simulink subsystem "Controller_Sub"  (R2024a)
settings: Solver=VariableStepAuto  StartTime=0.0  StopTime=10.0  RelTol=1e-3
undefined symbols (not defined in the file): body_inertia, body_mass, Dinv, DiscIntNeverNeededParam, Dmat, motor_gyration, motor_resistance, nominal_voltage, pwm_limit, torque_limit, wheel_distance, wheel_radius
libraries: slpidlib x2, dspfdesign x2
settings Model: Creator=Marij  LastModifiedBy=Marij

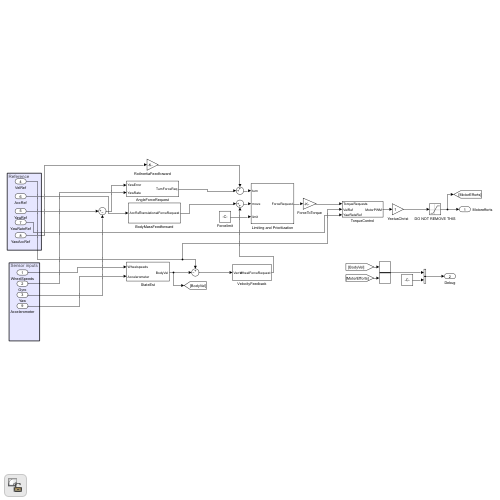
[thumbnail: Simulink's stored preview of the top-level diagram]
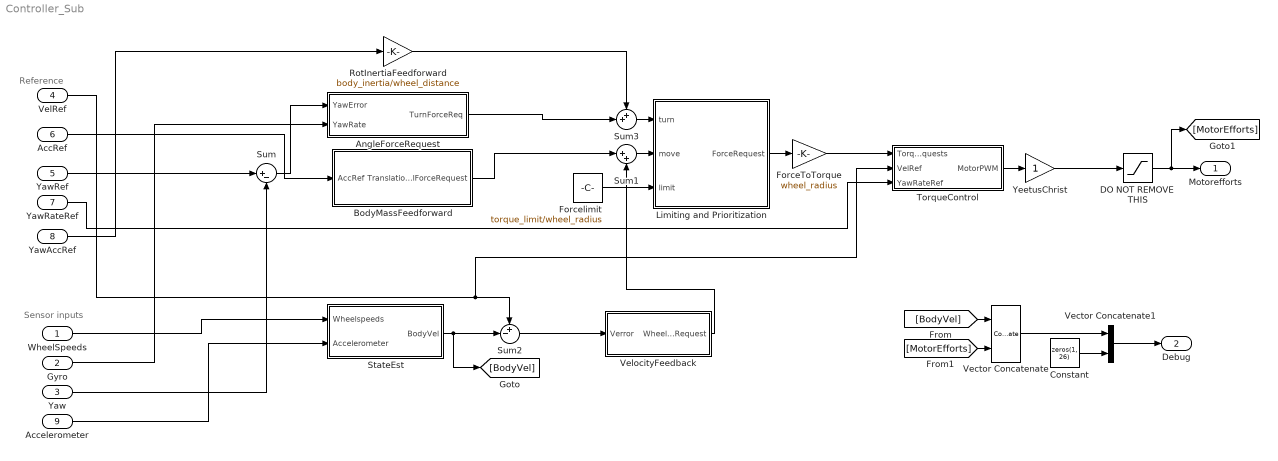
== system Controller_Sub ==
  note: Reference
  note: Sensor inputs
  WheelSpeeds : Inport  OutDataTypeStr=single  Unit=rad/s  PortDimensions=4  LockScale=on
  Gyro : Inport  Port=2  OutDataTypeStr=single  Unit=rad/s  PortDimensions=1
  Yaw : Inport  Port=3  OutDataTypeStr=single  Unit=rad  PortDimensions=1
  VelRef : Inport  Port=4  OutDataTypeStr=single  Unit=m/s  PortDimensions=2
  YawRef : Inport  Port=5
  AccRef : Inport  Port=6  OutDataTypeStr=single  Unit=m/s^2  PortDimensions=2
  YawRateRef : Inport  Port=7  OutDataTypeStr=single  Unit=rad/s
  YawAccRef : Inport  Port=8  OutDataTypeStr=single  Unit=rad/s^2
  Accelerometer : Inport  Port=9  OutDataTypeStr=single  Unit=m/s^2  PortDimensions=2
  AngleForceRequest : Subsystem
  BodyMassFeedforward : Subsystem
  Constant : Constant  Value=zeros(1, 26)  OutDataTypeStr=single
  DO NOT REMOVE THIS : Saturate  UpperLimit=pwm_limit  LowerLimit=-pwm_limit
  ForceToTorque : Gain  Gain=wheel_radius
  Forcelimit : Constant  Value=torque_limit/wheel_radius
  Limiting and Prioritization : Subsystem
  RotInertiaFeedforward : Gain  Gain=body_inertia/wheel_distance
  StateEst : Subsystem
  Sum : Sum  Inputs=|+-
  Sum1 : Sum  Inputs=|++
  Sum2 : Sum  Inputs=+-|
  Sum3 : Sum  Inputs=++|
  TorqueControl : Subsystem
  Vector Concatenate : Concatenate
  Vector Concatenate1 : Concatenate
  VelocityFeedback : Subsystem
  YeetusChrist : Gain
  Motorefforts : Outport  OutDataTypeStr=single  PortDimensions=4
  Debug : Outport  Port=2  OutDataTypeStr=single  PortDimensions=32
  wires:
  YeetusChrist/1 -> DO NOT REMOVE THIS/1
  Gyro/1 -> AngleForceRequest/2(YawRate)
  AccRef/1 -> BodyMassFeedforward/1(AccRef)
  Sum/1 -> AngleForceRequest/1(YawError)
  Accelerometer/1 -> StateEst/2(Accelerometer)
  StateEst/1(BodyVel) -> Sum2/2, [BodyVel]
  Sum3/1 -> Limiting and Prioritization/1(turn)
  YawRef/1 -> Sum/1
  TorqueControl/1(MotorPWM) -> YeetusChrist/1
  WheelSpeeds/1 -> StateEst/1(Wheelspeeds)
  Limiting and Prioritization/1(ForceRequest) -> ForceToTorque/1
  DO NOT REMOVE THIS/1 -> [MotorEfforts], Motorefforts/1
  Sum2/1 -> VelocityFeedback/1(Verror)
  [BodyVel] -> Vector Concatenate/1
  Yaw/1 -> Sum/2
  RotInertiaFeedforward/1 -> Sum3/1
  [MotorEfforts] -> Vector Concatenate/2
  VelocityFeedback/1(WheelForceRequest) -> Sum1/2
  Vector Concatenate1/1 -> Debug/1
  YawAccRef/1 -> RotInertiaFeedforward/1
  Vector Concatenate/1 -> Vector Concatenate1/1
  VelRef/1 -> TorqueControl/2(VelRef), Sum2/1
  BodyMassFeedforward/1(TranslationalForceRequest) -> Sum1/1
  YawRateRef/1 -> TorqueControl/3(YawRateRef)
  AngleForceRequest/1(TurnForceReq) -> Sum3/2
  ForceToTorque/1 -> TorqueControl/1(TorqueRequests)
  Sum1/1 -> Limiting and Prioritization/2(move)
  Constant/1 -> Vector Concatenate1/2
  Forcelimit/1 -> Limiting and Prioritization/3(limit)

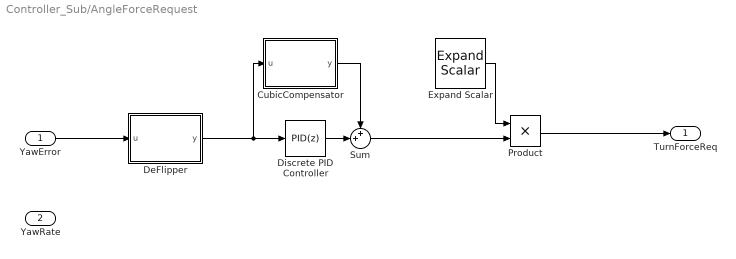
== system Controller_Sub/AngleForceRequest ==
  YawError : Inport  Unit=rad
  YawRate : Inport  Port=2
  CubicCompensator : MATLAB Function  TreatAsAtomicUnit=on
  DeFlipper : MATLAB Function  TreatAsAtomicUnit=on
  Discrete PID Controller : slpidlib/PID Controller  Controller=PID  Form=Parallel  TimeDomain=Discrete-time  UseExternalTs=off  SampleTime=-1  IntegratorMethod=Trapezoidal  FilterMethod=Trapezoidal  ControllerParametersSource=internal  P=9.0  I=0.1  UseKiTs=off  D=0.8  UseExternalDerivativeSource=off  N=100  UseFilter=on  TunerSelectOption=Transfer Function Based (PID Tuner App)  InitialConditionSource=internal  InitialConditionForIntegrator=0  InitialConditionForFilter=0  DifferentiatorICPrevScaledInput=0  ExternalReset=none  TrackingMode=off  Kt=1  LimitOutput=off  SatLimitsSource=internal  UpperSaturationLimit=inf  LowerSaturationLimit=-inf  LinearizeAsGain=off  AntiWindupMode=none  Kb=1  LimitIntegrator=off  UpperIntegratorSaturationLimit=inf  LowerIntegratorSaturationLimit=-inf  POutMin=[]  POutMax=[]  IOutMin=[]  IOutMax=[]  DOutMin=[]  DOutMax=[]  NOutMin=[]  NOutMax=[]  SumOutMin=[]  SumOutMax=[]  SaturationOutMin=[]  SaturationOutMax=[]  PParamMin=[]  PParamMax=[]  IParamMin=[]  IParamMax=[]  DParamMin=[]  DParamMax=[]  NParamMin=[]  NParamMax=[]  KbParamMin=[]  KbParamMax=[]  KtParamMin=[]  KtParamMax=[]  KbOutMin=[]  KbOutMax=[]  KtOutMin=[]  KtOutMax=[]  IntegratorOutMin=[]  IntegratorOutMax=[]  FilterOutMin=[]  FilterOutMax=[]  SumI1OutMin=[]  SumI1OutMax=[]  SumI2OutMin=[]  SumI2OutMax=[]  SumI3OutMin=[]  SumI3OutMax=[]  SumI4OutMin=[]  SumI4OutMax=[]  SumDOutMin=[]  SumDOutMax=[]  DifferentiatorOutMin=[]  DifferentiatorOutMax=[]  FilterDiffOutCoefMin=[]  FilterDiffOutCoefMax=[]  ReciprocalOutMin=[]  ReciprocalOutMax=[]  SumDenOutMin=[]  SumDenOutMax=[]  SumNumOutMin=[]  SumNumOutMax=[]  DivideOutMin=[]  DivideOutMax=[]  UdiffTsProdOutMin=[]  UdiffTsProdOutMax=[]  NTsProdOutMin=[]  NTsProdOutMax=[]  UintegralTsProdOutMin=[]  UintegralTsProdOutMax=[]  UngainTsProdOutMin=[]  UngainTsProdOutMax=[]  ClampingZeroOutDataTypeStr=Inherit: Inherit via back propagation  ClampingZeroOutMin=[]  ClampingZeroOutMax=[]  FilterDenConstantOutDataTypeStr=Inherit: Inherit via back propagation  FilterDenConstantOutMin=[]  FilterDenConstantOutMax=[]  PCopyOutDataTypeStr=Inherit: Inherit via back propagation  PCopyOutMin=[]  PCopyOutMax=[]  NCopyOutDataTypeStr=Inherit: Inherit via back propagation  NCopyOutMin=[]  NCopyOutMax=[]  IntegratorContinuousStateAttributes=''  IntegratorStateMustResolveToSignalObject=off  IntegratorRTWStateStorageClass=Auto  FilterContinuousStateAttributes=''  FilterStateMustResolveToSignalObject=off  FilterRTWStateStorageClass=Auto  ParallelPVariant=InternalParameters  IdealPVariant=Disabled  IVariant=InternalParameters  DVariant=InternalParameters  IntegratorVariant=Discrete  SatVariant=Disabled  AWVariant=Passthrough  PCopyVariant=Disabled  TRVariant=Disabled  FdbkBlocksVariant=Forward  IdealPFdbkVariant=Disabled  SatFdbkVariant=Disabled  DerivativeFilterVariant=TrapezoidalFilter  NVariant=InternalParameters  NCopyVariant=InternalParameters  FilterICVariant=InternalICsFilter  IntegratorICVariant=InternalICs  ExternalResetVariant=Disabled  TRSumVariant=Passthrough  SumFdbkVariant=Disabled  SumVariant=Sum_PID  TsampFilterVariant=InternalTs  TsampNgainVariant=Passthrough  TsampIntegralVariant=Disabled_SignalSpec  ExternalSaturationOutDataTypeStr=Inherit: Same as second input  DerivativeSourceVariant=ErrorSignal
      settings: LibrarySourceBlock=simulink/Discrete/Discrete PID Controller
  Expand Scalar : ExpandScalar  OutputDimensions=4  OutDataTypeStr=single  SampleTime=-1
  Product : Product  OutDataTypeStr=single
  Sum : Sum  Inputs=++|
  TurnForceReq : Outport  Unit=N
  wires:
  Sum/1 -> Product/2
  CubicCompensator/1(y) -> Sum/1
  Discrete PID Controller/1 -> Sum/2
  DeFlipper/1(y) -> Discrete PID Controller/1, CubicCompensator/1(u)
  YawError/1 -> DeFlipper/1(u)
  Product/1 -> TurnForceReq/1
  Expand Scalar/1 -> Product/1

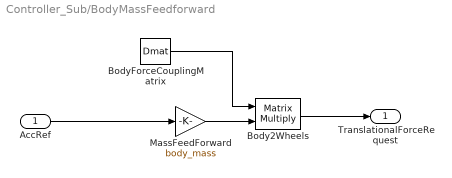
== system Controller_Sub/BodyMassFeedforward ==
  AccRef : Inport
  Body2Wheels : Product  Multiplication=Matrix(*)
  BodyForceCouplingMatrix : Constant  Value=Dmat  VectorParams1D=off  OutDataTypeStr=single
  MassFeedForward : Gain  Gain=body_mass
  TranslationalForceRequest : Outport  Unit=N
  wires:
  AccRef/1 -> MassFeedForward/1
  Body2Wheels/1 -> TranslationalForceRequest/1
  MassFeedForward/1 -> Body2Wheels/2
  BodyForceCouplingMatrix/1 -> Body2Wheels/1

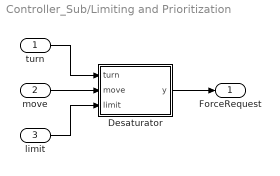
== system Controller_Sub/Limiting and Prioritization ==
  turn : Inport  Unit=N  PortDimensions=4
  move : Inport  Port=2  Unit=N  PortDimensions=4
  limit : Inport  Port=3  Unit=N
  Desaturator : MATLAB Function  TreatAsAtomicUnit=on
  ForceRequest : Outport  Unit=N  PortDimensions=4
  wires:
  Desaturator/1(y) -> ForceRequest/1
  turn/1 -> Desaturator/1(turn)
  move/1 -> Desaturator/2(move)
  limit/1 -> Desaturator/3(limit)

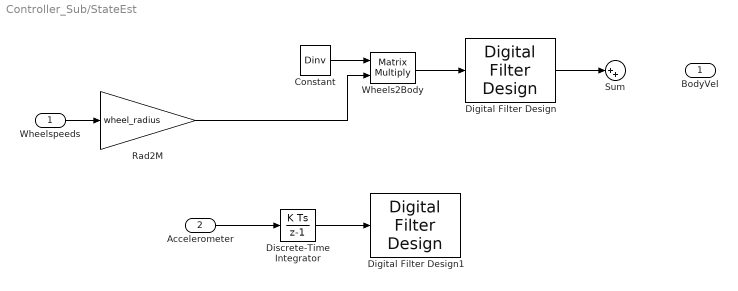
== system Controller_Sub/StateEst ==
  Wheelspeeds : Inport
  Accelerometer : Inport  Port=2  Unit=m/s^2  PortDimensions=2
  Constant : Constant  Value=Dinv
  Digital Filter Design : dspfdesign/Digital Filter Design  mwdsp_browser_bugfix_var=off
  Digital Filter Design1 : dspfdesign/Digital Filter Design  mwdsp_browser_bugfix_var=off
  Discrete-Time Integrator : DiscreteIntegrator  SampleTime=-1  ICPrevOutput=DiscIntNeverNeededParam  ICPrevScaledInput=DiscIntNeverNeededParam
  Rad2M : Gain  Gain=wheel_radius
  Sum : Sum  Inputs=|++
  Wheels2Body : Product  Multiplication=Matrix(*)
  BodyVel : Outport  Unit=m/s  PortDimensions=2
  wires:
  Wheelspeeds/1 -> Rad2M/1
  Digital Filter Design/1 -> Sum/1
  Wheels2Body/1 -> Digital Filter Design/1
  Discrete-Time Integrator/1 -> Digital Filter Design1/1
  Accelerometer/1 -> Discrete-Time Integrator/1
  Constant/1 -> Wheels2Body/1
  Rad2M/1 -> Wheels2Body/2

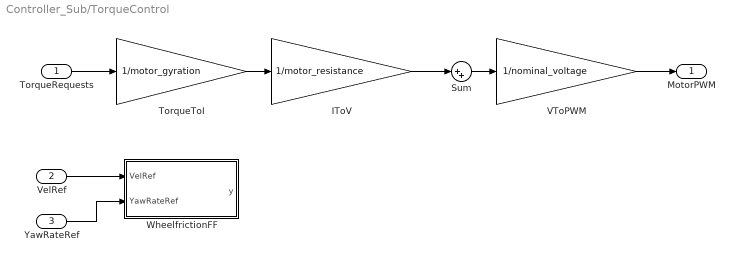
== system Controller_Sub/TorqueControl ==
  TorqueRequests : Inport
  VelRef : Inport  Port=2
  YawRateRef : Inport  Port=3
  IToV : Gain  Gain=1/motor_resistance
  Sum : Sum  Inputs=|++
  TorqueToI : Gain  Gain=1/motor_gyration
  VToPWM : Gain  Gain=1/nominal_voltage
  WheelfrictionFF : Subsystem
  MotorPWM : Outport
  wires:
  TorqueToI/1 -> IToV/1
  VToPWM/1 -> MotorPWM/1
  VelRef/1 -> WheelfrictionFF/1(VelRef)
  YawRateRef/1 -> WheelfrictionFF/2(YawRateRef)
  TorqueRequests/1 -> TorqueToI/1
  IToV/1 -> Sum/1
  Sum/1 -> VToPWM/1

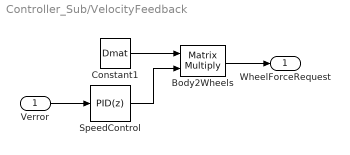
== system Controller_Sub/VelocityFeedback ==
  Verror : Inport  Unit=m/s  PortDimensions=2
  Body2Wheels : Product  Multiplication=Matrix(*)
  Constant1 : Constant  Value=Dmat
  SpeedControl : slpidlib/PID Controller  Controller=PID  Form=Parallel  TimeDomain=Discrete-time  UseExternalTs=off  SampleTime=-1  IntegratorMethod=Forward Euler  FilterMethod=Forward Euler  ControllerParametersSource=internal  P=10  I=0  UseKiTs=off  D=0  UseExternalDerivativeSource=off  N=100  UseFilter=on  TunerSelectOption=Transfer Function Based (PID Tuner App)  InitialConditionSource=internal  InitialConditionForIntegrator=0  InitialConditionForFilter=0  DifferentiatorICPrevScaledInput=0  ExternalReset=none  TrackingMode=off  Kt=1  LimitOutput=off  SatLimitsSource=internal  UpperSaturationLimit=inf  LowerSaturationLimit=-inf  LinearizeAsGain=off  AntiWindupMode=none  Kb=1  LimitIntegrator=off  UpperIntegratorSaturationLimit=inf  LowerIntegratorSaturationLimit=-inf  POutMin=[]  POutMax=[]  IOutMin=[]  IOutMax=[]  DOutMin=[]  DOutMax=[]  NOutMin=[]  NOutMax=[]  SumOutMin=[]  SumOutMax=[]  SaturationOutMin=[]  SaturationOutMax=[]  PParamMin=[]  PParamMax=[]  IParamMin=[]  IParamMax=[]  DParamMin=[]  DParamMax=[]  NParamMin=[]  NParamMax=[]  KbParamMin=[]  KbParamMax=[]  KtParamMin=[]  KtParamMax=[]  KbOutMin=[]  KbOutMax=[]  KtOutMin=[]  KtOutMax=[]  IntegratorOutMin=[]  IntegratorOutMax=[]  FilterOutMin=[]  FilterOutMax=[]  SumI1OutMin=[]  SumI1OutMax=[]  SumI2OutMin=[]  SumI2OutMax=[]  SumI3OutMin=[]  SumI3OutMax=[]  SumI4OutMin=[]  SumI4OutMax=[]  SumDOutMin=[]  SumDOutMax=[]  DifferentiatorOutMin=[]  DifferentiatorOutMax=[]  FilterDiffOutCoefMin=[]  FilterDiffOutCoefMax=[]  ReciprocalOutMin=[]  ReciprocalOutMax=[]  SumDenOutMin=[]  SumDenOutMax=[]  SumNumOutMin=[]  SumNumOutMax=[]  DivideOutMin=[]  DivideOutMax=[]  UdiffTsProdOutMin=[]  UdiffTsProdOutMax=[]  NTsProdOutMin=[]  NTsProdOutMax=[]  UintegralTsProdOutMin=[]  UintegralTsProdOutMax=[]  UngainTsProdOutMin=[]  UngainTsProdOutMax=[]  ClampingZeroOutDataTypeStr=Inherit: Inherit via back propagation  ClampingZeroOutMin=[]  ClampingZeroOutMax=[]  FilterDenConstantOutDataTypeStr=Inherit: Inherit via back propagation  FilterDenConstantOutMin=[]  FilterDenConstantOutMax=[]  PCopyOutDataTypeStr=Inherit: Inherit via back propagation  PCopyOutMin=[]  PCopyOutMax=[]  NCopyOutDataTypeStr=Inherit: Inherit via back propagation  NCopyOutMin=[]  NCopyOutMax=[]  IntegratorContinuousStateAttributes=''  IntegratorStateMustResolveToSignalObject=off  IntegratorRTWStateStorageClass=Auto  FilterContinuousStateAttributes=''  FilterStateMustResolveToSignalObject=off  FilterRTWStateStorageClass=Auto  ParallelPVariant=InternalParameters  IdealPVariant=Disabled  IVariant=InternalParameters  DVariant=InternalParameters  IntegratorVariant=Discrete  SatVariant=Disabled  AWVariant=Passthrough  PCopyVariant=Disabled  TRVariant=Disabled  FdbkBlocksVariant=Forward  IdealPFdbkVariant=Disabled  SatFdbkVariant=Disabled  DerivativeFilterVariant=ForwardEulerFilter  NVariant=InternalParameters  NCopyVariant=Disabled  FilterICVariant=InternalICsFilter  IntegratorICVariant=InternalICs  ExternalResetVariant=Disabled  TRSumVariant=Passthrough  SumFdbkVariant=Disabled  SumVariant=Sum_PID  TsampFilterVariant=InternalTs  TsampNgainVariant=Passthrough  TsampIntegralVariant=Disabled_SignalSpec  ExternalSaturationOutDataTypeStr=Inherit: Same as second input  DerivativeSourceVariant=ErrorSignal
      settings: LibrarySourceBlock=simulink/Discrete/Discrete PID Controller
  WheelForceRequest : Outport  Unit=N  PortDimensions=4
  wires:
  Body2Wheels/1 -> WheelForceRequest/1
  SpeedControl/1 -> Body2Wheels/2
  Constant1/1 -> Body2Wheels/1
  Verror/1 -> SpeedControl/1

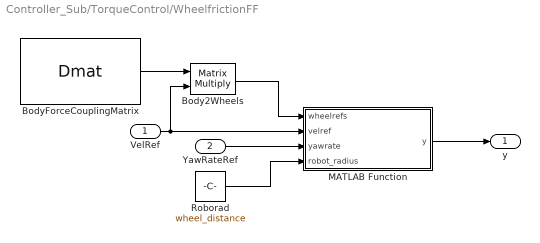
== system Controller_Sub/TorqueControl/WheelfrictionFF ==
  VelRef : Inport  PortDimensions=2
  YawRateRef : Inport  Port=2  PortDimensions=1
  Body2Wheels : Product  Multiplication=Matrix(*)
  BodyForceCouplingMatrix : Constant  Value=Dmat  VectorParams1D=off  OutDataTypeStr=single
  MATLAB Function : MATLAB Function  TreatAsAtomicUnit=on
  Roborad : Constant  Value=wheel_distance
  y : Outport  PortDimensions=4
  wires:
  MATLAB Function/1(y) -> y/1
  Roborad/1 -> MATLAB Function/4(robot_radius)
  YawRateRef/1 -> MATLAB Function/3(yawrate)
  Body2Wheels/1 -> MATLAB Function/1(wheelrefs)
  VelRef/1 -> Body2Wheels/2, MATLAB Function/2(velref)
  BodyForceCouplingMatrix/1 -> Body2Wheels/1

== matlab function Controller_Sub/Limiting and Prioritization/Desaturator ==
  data: turn input; y output; move input; limit input
function y = fcn(turn, move, limit)
y = turn_prio_desaturator(turn, move, limit);
end

== matlab function Controller_Sub/AngleForceRequest/DeFlipper ==
  data: u input; y output
function y = fcn(u)

y = limit_angle(u);

== matlab function Controller_Sub/TorqueControl/WheelfrictionFF/MATLAB Function ==
  data: wheelrefs input; velref input; yawrate input; robot_radius input; y output
function y=fcn(wheelrefs, velref, yawrate, robot_radius)
[theta, rho] = cart2pol(velref(1), velref(2));
y = friction_feedforward(wheelrefs', rho, theta, yawrate, robot_radius)';
end

== matlab function Controller_Sub/AngleForceRequest/CubicCompensator ==
  data: u input; y output
function y = fcn(u)

y = 100.0*u^3;
